simulink model "MotorLink"  (R2020b)
settings: Solver=ode4  StartTime=0.0  StopTime=15  FixedStep=0.001  RelTol=1e-3
values from neighbouring files (symbols this model uses):
  A = [0 1 0; -m*l*g/den -d/den km/den; 0 -ke/L -R/L]    [init_MotorLink.m]
  A_dist = [A_dist; [0 0 0 0]]    [init_MotorLink.m]
  B = [0 0 1/L]'    [init_MotorLink.m]
  B_dist = [B;0]    [init_MotorLink.m]
  C = [1 0 0]    [init_MotorLink.m]
  C_dist = [C,0]    [init_MotorLink.m]
  d = 0.1    [init_MotorLink.m]
  g = 9.81    [init_MotorLink.m]
  h = place(A', C', q)'    [init_MotorLink.m]
  h_dist = place(A_dist', C_dist', q_dist)'    [init_MotorLink.m]
  J = 0.001    [init_MotorLink.m]
  k = kR * inv(T)    [init_MotorLink.m]
  ke = 0.1    [init_MotorLink.m]
  km = 0.1    [init_MotorLink.m]
  L = 0.01    [init_MotorLink.m]
  l = 0.1375    [init_MotorLink.m]
  m = 1    [init_MotorLink.m]
  R = 0.1    [init_MotorLink.m]
settings Model: Creator=baradaran  LastModifiedBy=jsol

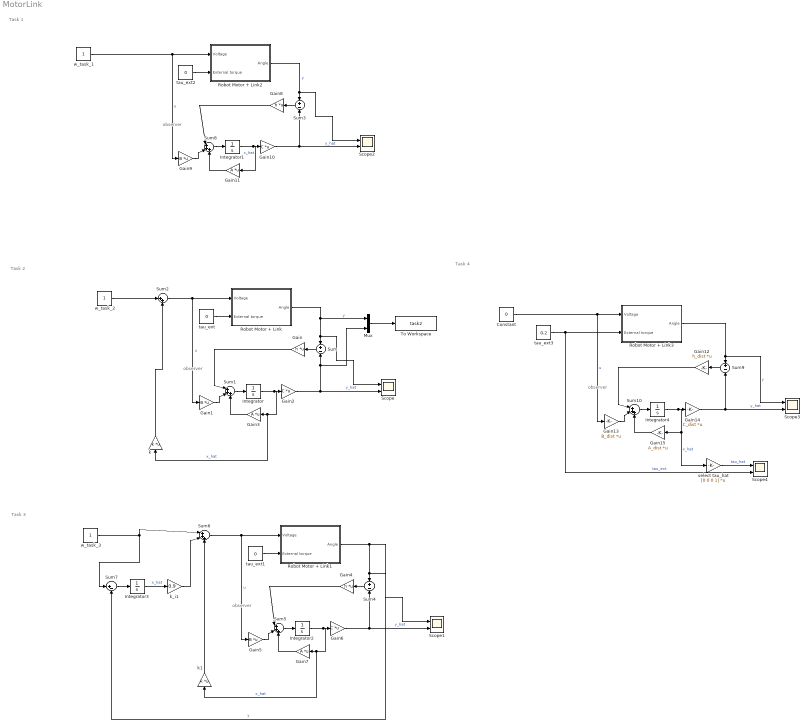
== system MotorLink ==
  note: Task 4
  note: Task 3
  note: Task 2
  note: Task 1
  note: observer
  note: observer
  note: observer
  note: observer
  Constant : Constant  Value=0
  Gain : Gain  Gain=h  Multiplication=Matrix(K*u)
  Gain1 : Gain  Gain=B  Multiplication=Matrix(K*u)
  Gain10 : Gain  Gain=C  Multiplication=Matrix(K*u)
  Gain11 : Gain  Gain=A  Multiplication=Matrix(K*u)
  Gain12 : Gain  Gain=h_dist  Multiplication=Matrix(K*u)
  Gain13 : Gain  Gain=B_dist  Multiplication=Matrix(K*u)
  Gain14 : Gain  Gain=C_dist  Multiplication=Matrix(K*u)
  Gain15 : Gain  Gain=A_dist  Multiplication=Matrix(K*u)
  Gain2 : Gain  Gain=C  Multiplication=Matrix(K*u)
  Gain3 : Gain  Gain=A  Multiplication=Matrix(K*u)
  Gain4 : Gain  Gain=h  Multiplication=Matrix(K*u)
  Gain5 : Gain  Gain=B  Multiplication=Matrix(K*u)
  Gain6 : Gain  Gain=C  Multiplication=Matrix(K*u)
  Gain7 : Gain  Gain=A  Multiplication=Matrix(K*u)
  Gain8 : Gain  Gain=h  Multiplication=Matrix(K*u)
  Gain9 : Gain  Gain=B  Multiplication=Matrix(K*u)
  Integrator{,1..4} (5 alike) : Integrator
  Mux : Mux  Inputs=2
  Robot Motor + Link : Subsystem  mask{J=J, ke=ke, R=R, In=L, km=km, d=d, m=m, l=l, g=g}
      mask prompts: J "Massenträgheitsmoment"; ke "elektrische Motorkonstante"; R "elektrischer Widerstand"; In "Induktivität"; km "mechanische Motorkonstante"; d "mechanische Dämpfung"; m "Gelenkmasse"; l "Massenschwerpunkt des Gelenks"; g "Gravitation"
  Robot Motor + Link1 : Subsystem  mask{J=J, ke=ke, R=R, In=L, km=km, d=d, m=m, l=l, g=g}
      mask prompts: J "Massenträgheitsmoment"; ke "elektrische Motorkonstante"; R "elektrischer Widerstand"; In "Induktivität"; km "mechanische Motorkonstante"; d "mechanische Dämpfung"; m "Gelenkmasse"; l "Massenschwerpunkt des Gelenks"; g "Gravitation"
  Robot Motor + Link2 : Subsystem  mask{J=J, ke=ke, R=R, In=L, km=km, d=d, m=m, l=l, g=g}
      mask prompts: J "Massenträgheitsmoment"; ke "elektrische Motorkonstante"; R "elektrischer Widerstand"; In "Induktivität"; km "mechanische Motorkonstante"; d "mechanische Dämpfung"; m "Gelenkmasse"; l "Massenschwerpunkt des Gelenks"; g "Gravitation"
  Robot Motor + Link3 : Subsystem  mask{J=J, ke=ke, R=R, In=L, km=km, d=d, m=m, l=l, g=g}
      mask prompts: J "Massenträgheitsmoment"; ke "elektrische Motorkonstante"; R "elektrischer Widerstand"; In "Induktivität"; km "mechanische Motorkonstante"; d "mechanische Dämpfung"; m "Gelenkmasse"; l "Massenschwerpunkt des Gelenks"; g "Gravitation"
  Scope{,1..4} (5 alike) : Scope  NumInputPorts=2
  Sum{,3..4,9} (4 alike) : Sum  Inputs=+|-
  Sum{1,5..6,8,10} (5 alike) : Sum  Inputs=|+++
  Sum2 : Sum  Inputs=|++
  Sum7 : Sum  Inputs=|+-
  To Workspace : ToWorkspace  VariableName=task2  SaveFormat=Timeseries  SampleTime=-1
  k : Gain  Gain=k  Multiplication=Matrix(K*u)
  k1 : Gain  Gain=k  Multiplication=Matrix(K*u)
  k_i1 : Gain  Gain=0.9
  select tau_hat : Gain  Gain=[0 0 0 1]  Multiplication=Matrix(K*u)
  tau_ext : Constant  Value=0
  tau_ext1 : Constant  Value=0
  tau_ext2 : Constant  Value=0
  tau_ext3 : Constant  Value=0.2
  w_task_1 : Constant
  w_task_2 : Constant
  w_task_3 : Constant
  wires:
  w_task_2/1 -> Sum2/1
  tau_ext/1 -> Robot Motor + Link/2(External torque)
  Robot Motor + Link/1(Angle) -> Mux/1, Scope/1, Sum/1  "y"
  Gain2/1 -> Scope/2, Mux/2, Sum/2  "y_hat"
  Sum/1 -> Gain/1
  Gain/1 -> Sum1/1
  Gain1/1 -> Sum1/2
  Sum1/1 -> Integrator/1
  Integrator/1 -> k/1, Gain3/1, Gain2/1  "x_hat"
  Gain3/1 -> Sum1/3
  Sum2/1 -> Gain1/1, Robot Motor + Link/1(Voltage)  "u"
  Gain5/1 -> Sum5/2
  Sum4/1 -> Gain4/1
  Gain7/1 -> Sum5/3
  Gain6/1 -> Scope1/2, Sum4/2  "y_hat"
  Sum7/1 -> Integrator3/1
  k1/1 -> Sum6/3
  Integrator2/1 -> k1/1, Gain7/1, Gain6/1  "x_hat"
  Gain4/1 -> Sum5/1
  Robot Motor + Link1/1(Angle) -> Sum7/2, Scope1/1, Sum4/1  "y"
  Sum5/1 -> Integrator2/1
  Integrator3/1 -> k_i1/1  "x_hat"
  w_task_3/1 -> Sum7/1, Sum6/1
  k_i1/1 -> Sum6/2
  tau_ext1/1 -> Robot Motor + Link1/2(External torque)
  Sum6/1 -> Gain5/1, Robot Motor + Link1/1(Voltage)  "u"
  k/1 -> Sum2/2
  Gain9/1 -> Sum8/2
  Sum3/1 -> Gain8/1
  Gain11/1 -> Sum8/3
  Gain10/1 -> Scope2/2, Sum3/2  "y_hat"
  Integrator1/1 -> Gain11/1, Gain10/1  "x_hat"
  Gain8/1 -> Sum8/1
  Sum8/1 -> Integrator1/1
  Robot Motor + Link2/1(Angle) -> Scope2/1, Sum3/1  "y"
  tau_ext2/1 -> Robot Motor + Link2/2(External torque)
  w_task_1/1 -> Gain9/1, Robot Motor + Link2/1(Voltage)  "u"
  tau_ext3/1 -> Robot Motor + Link3/2(External torque), Scope4/2  "tau_ext"
  Gain13/1 -> Sum10/2
  Sum9/1 -> Gain12/1
  Robot Motor + Link3/1(Angle) -> Scope3/1, Sum9/1  "y"
  Constant/1 -> Gain13/1, Robot Motor + Link3/1(Voltage)  "u"
  Gain15/1 -> Sum10/3
  Gain14/1 -> Scope3/2, Sum9/2  "y_hat"
  Integrator4/1 -> select tau_hat/1, Gain15/1, Gain14/1  "x_hat"
  Gain12/1 -> Sum10/1
  Sum10/1 -> Integrator4/1
  select tau_hat/1 -> Scope4/1  "tau_hat"
  Mux/1 -> To Workspace/1

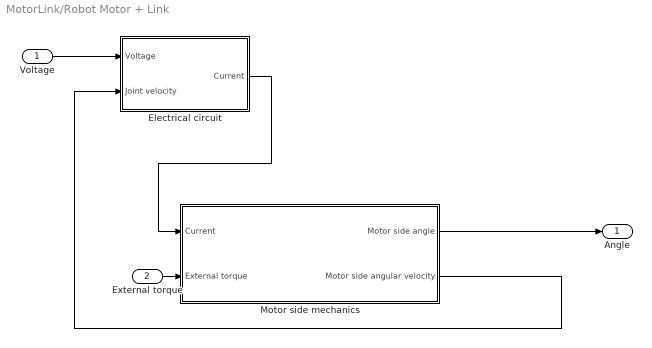
== system MotorLink/Robot Motor + Link ==
  Voltage : Inport
  External torque : Inport  Port=2
  Electrical circuit : Subsystem
  Motor side mechanics : Subsystem
  Angle : Outport  VectorParamsAs1DForOutWhenUnconnected=off
  wires:
  External torque/1 -> Motor side mechanics/2(External torque)
  Motor side mechanics/1(Motor side angle) -> Angle/1
  Motor side mechanics/2(Motor side angular velocity) -> Electrical circuit/2(Joint velocity)
  Electrical circuit/1(Current) -> Motor side mechanics/1(Current)
  Voltage/1 -> Electrical circuit/1(Voltage)

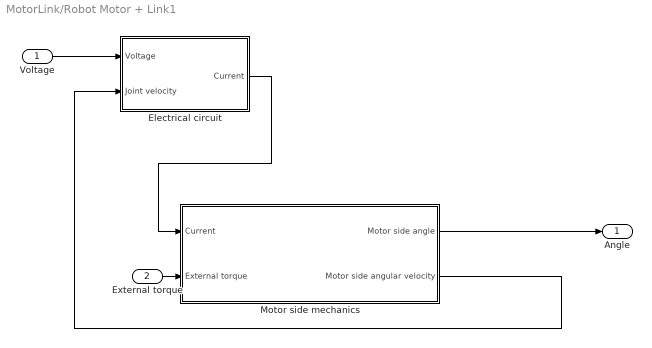
== system MotorLink/Robot Motor + Link1 ==
  Voltage : Inport
  External torque : Inport  Port=2
  Electrical circuit : Subsystem
  Motor side mechanics : Subsystem
  Angle : Outport  VectorParamsAs1DForOutWhenUnconnected=off
  wires:
  External torque/1 -> Motor side mechanics/2(External torque)
  Motor side mechanics/1(Motor side angle) -> Angle/1
  Motor side mechanics/2(Motor side angular velocity) -> Electrical circuit/2(Joint velocity)
  Electrical circuit/1(Current) -> Motor side mechanics/1(Current)
  Voltage/1 -> Electrical circuit/1(Voltage)

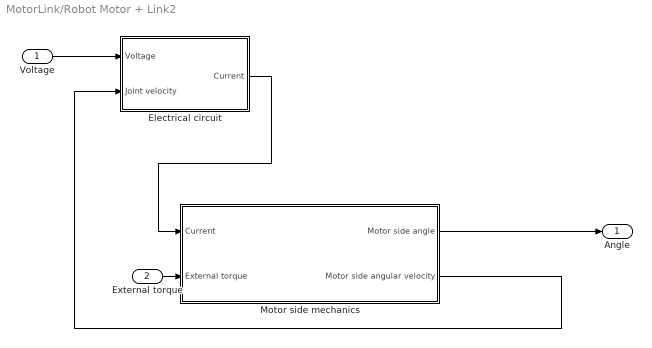
== system MotorLink/Robot Motor + Link2 ==
  Voltage : Inport
  External torque : Inport  Port=2
  Electrical circuit : Subsystem
  Motor side mechanics : Subsystem
  Angle : Outport  VectorParamsAs1DForOutWhenUnconnected=off
  wires:
  External torque/1 -> Motor side mechanics/2(External torque)
  Motor side mechanics/1(Motor side angle) -> Angle/1
  Motor side mechanics/2(Motor side angular velocity) -> Electrical circuit/2(Joint velocity)
  Electrical circuit/1(Current) -> Motor side mechanics/1(Current)
  Voltage/1 -> Electrical circuit/1(Voltage)

== system MotorLink/Robot Motor + Link3 ==
  Voltage : Inport
  External torque : Inport  Port=2
  Electrical circuit : Subsystem
  Motor side mechanics : Subsystem
  Angle : Outport  VectorParamsAs1DForOutWhenUnconnected=off
  wires:
  External torque/1 -> Motor side mechanics/2(External torque)
  Motor side mechanics/1(Motor side angle) -> Angle/1
  Motor side mechanics/2(Motor side angular velocity) -> Electrical circuit/2(Joint velocity)
  Electrical circuit/1(Current) -> Motor side mechanics/1(Current)
  Voltage/1 -> Electrical circuit/1(Voltage)

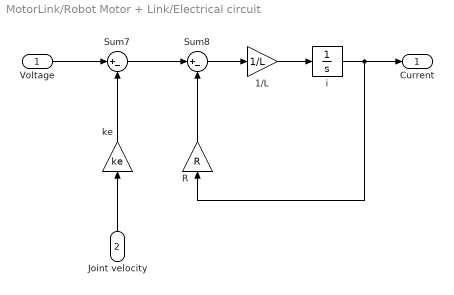
== system MotorLink/Robot Motor + Link/Electrical circuit ==
  Voltage : Inport
  Joint velocity : Inport  Port=2
  1/L : Gain  Gain=1/L
  R : Gain  Gain=R
  Sum7 : Sum  Inputs=|+-
  Sum8 : Sum  Inputs=|+-
  i : Integrator
  ke : Gain  Gain=ke
  Current : Outport  VectorParamsAs1DForOutWhenUnconnected=off
  wires:
  Sum7/1 -> Sum8/1
  i/1 -> R/1, Current/1
  R/1 -> Sum8/2
  Voltage/1 -> Sum7/1
  Joint velocity/1 -> ke/1
  ke/1 -> Sum7/2
  Sum8/1 -> 1/L/1
  1/L/1 -> i/1

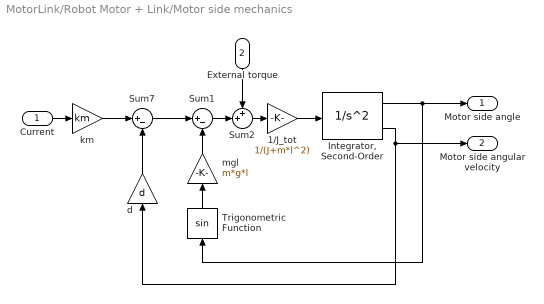
== system MotorLink/Robot Motor + Link/Motor side mechanics ==
  Current : Inport
  External torque : Inport  Port=2
  1/J_tot : Gain  Gain=1/(J+m*l^2)
  "Integrator, Second-Order" : SecondOrderIntegrator
  Sum1 : Sum  Inputs=|+-
  Sum2 : Sum  Inputs=++|
  Sum7 : Sum  Inputs=|+-
  Trigonometric Function : Trigonometry
  d : Gain  Gain=d
  km : Gain  Gain=km
  mgl : Gain  Gain=m*g*l
  Motor side angle : Outport  VectorParamsAs1DForOutWhenUnconnected=off
  Motor side angular velocity : Outport  Port=2  VectorParamsAs1DForOutWhenUnconnected=off
  wires:
  External torque/1 -> Sum2/1
  Sum1/1 -> Sum2/2
  Sum2/1 -> 1/J_tot/1
  Trigonometric Function/1 -> mgl/1
  Current/1 -> km/1
  "Integrator, Second-Order"/2 -> d/1, Motor side angular velocity/1
  1/J_tot/1 -> "Integrator, Second-Order"/1
  "Integrator, Second-Order"/1 -> Motor side angle/1, Trigonometric Function/1
  Sum7/1 -> Sum1/1
  mgl/1 -> Sum1/2
  d/1 -> Sum7/2
  km/1 -> Sum7/1

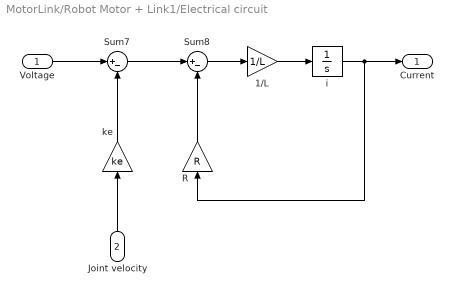
== system MotorLink/Robot Motor + Link1/Electrical circuit ==
  Voltage : Inport
  Joint velocity : Inport  Port=2
  1/L : Gain  Gain=1/L
  R : Gain  Gain=R
  Sum7 : Sum  Inputs=|+-
  Sum8 : Sum  Inputs=|+-
  i : Integrator
  ke : Gain  Gain=ke
  Current : Outport  VectorParamsAs1DForOutWhenUnconnected=off
  wires:
  Sum7/1 -> Sum8/1
  i/1 -> R/1, Current/1
  R/1 -> Sum8/2
  Voltage/1 -> Sum7/1
  Joint velocity/1 -> ke/1
  ke/1 -> Sum7/2
  Sum8/1 -> 1/L/1
  1/L/1 -> i/1

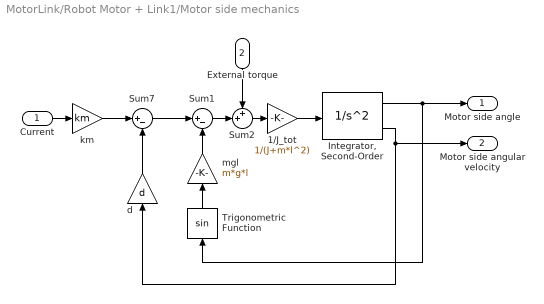
== system MotorLink/Robot Motor + Link1/Motor side mechanics ==
  Current : Inport
  External torque : Inport  Port=2
  1/J_tot : Gain  Gain=1/(J+m*l^2)
  "Integrator, Second-Order" : SecondOrderIntegrator
  Sum1 : Sum  Inputs=|+-
  Sum2 : Sum  Inputs=++|
  Sum7 : Sum  Inputs=|+-
  Trigonometric Function : Trigonometry
  d : Gain  Gain=d
  km : Gain  Gain=km
  mgl : Gain  Gain=m*g*l
  Motor side angle : Outport  VectorParamsAs1DForOutWhenUnconnected=off
  Motor side angular velocity : Outport  Port=2  VectorParamsAs1DForOutWhenUnconnected=off
  wires:
  External torque/1 -> Sum2/1
  Sum1/1 -> Sum2/2
  Sum2/1 -> 1/J_tot/1
  Trigonometric Function/1 -> mgl/1
  Current/1 -> km/1
  "Integrator, Second-Order"/2 -> d/1, Motor side angular velocity/1
  1/J_tot/1 -> "Integrator, Second-Order"/1
  "Integrator, Second-Order"/1 -> Motor side angle/1, Trigonometric Function/1
  Sum7/1 -> Sum1/1
  mgl/1 -> Sum1/2
  d/1 -> Sum7/2
  km/1 -> Sum7/1

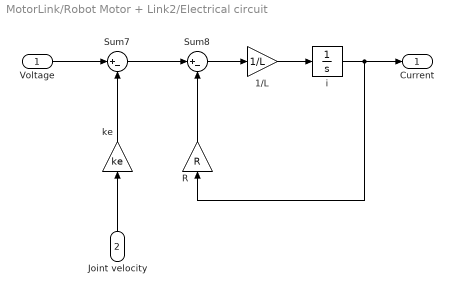
== system MotorLink/Robot Motor + Link2/Electrical circuit ==
  Voltage : Inport
  Joint velocity : Inport  Port=2
  1/L : Gain  Gain=1/L
  R : Gain  Gain=R
  Sum7 : Sum  Inputs=|+-
  Sum8 : Sum  Inputs=|+-
  i : Integrator
  ke : Gain  Gain=ke
  Current : Outport  VectorParamsAs1DForOutWhenUnconnected=off
  wires:
  Sum7/1 -> Sum8/1
  i/1 -> R/1, Current/1
  R/1 -> Sum8/2
  Voltage/1 -> Sum7/1
  Joint velocity/1 -> ke/1
  ke/1 -> Sum7/2
  Sum8/1 -> 1/L/1
  1/L/1 -> i/1

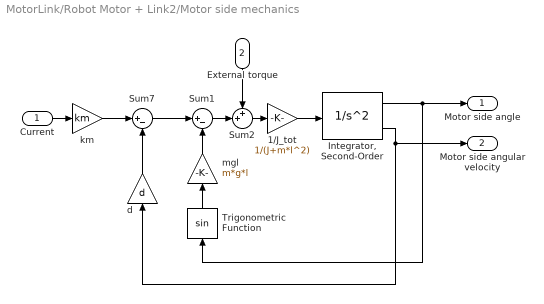
== system MotorLink/Robot Motor + Link2/Motor side mechanics ==
  Current : Inport
  External torque : Inport  Port=2
  1/J_tot : Gain  Gain=1/(J+m*l^2)
  "Integrator, Second-Order" : SecondOrderIntegrator
  Sum1 : Sum  Inputs=|+-
  Sum2 : Sum  Inputs=++|
  Sum7 : Sum  Inputs=|+-
  Trigonometric Function : Trigonometry
  d : Gain  Gain=d
  km : Gain  Gain=km
  mgl : Gain  Gain=m*g*l
  Motor side angle : Outport  VectorParamsAs1DForOutWhenUnconnected=off
  Motor side angular velocity : Outport  Port=2  VectorParamsAs1DForOutWhenUnconnected=off
  wires:
  External torque/1 -> Sum2/1
  Sum1/1 -> Sum2/2
  Sum2/1 -> 1/J_tot/1
  Trigonometric Function/1 -> mgl/1
  Current/1 -> km/1
  "Integrator, Second-Order"/2 -> d/1, Motor side angular velocity/1
  1/J_tot/1 -> "Integrator, Second-Order"/1
  "Integrator, Second-Order"/1 -> Motor side angle/1, Trigonometric Function/1
  Sum7/1 -> Sum1/1
  mgl/1 -> Sum1/2
  d/1 -> Sum7/2
  km/1 -> Sum7/1

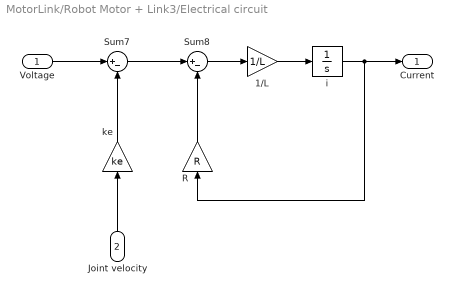
== system MotorLink/Robot Motor + Link3/Electrical circuit ==
  Voltage : Inport
  Joint velocity : Inport  Port=2
  1/L : Gain  Gain=1/L
  R : Gain  Gain=R
  Sum7 : Sum  Inputs=|+-
  Sum8 : Sum  Inputs=|+-
  i : Integrator
  ke : Gain  Gain=ke
  Current : Outport  VectorParamsAs1DForOutWhenUnconnected=off
  wires:
  Sum7/1 -> Sum8/1
  i/1 -> R/1, Current/1
  R/1 -> Sum8/2
  Voltage/1 -> Sum7/1
  Joint velocity/1 -> ke/1
  ke/1 -> Sum7/2
  Sum8/1 -> 1/L/1
  1/L/1 -> i/1

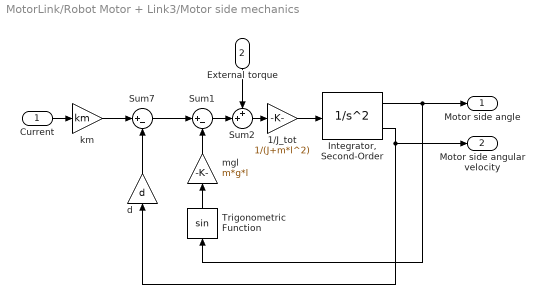
== system MotorLink/Robot Motor + Link3/Motor side mechanics ==
  Current : Inport
  External torque : Inport  Port=2
  1/J_tot : Gain  Gain=1/(J+m*l^2)
  "Integrator, Second-Order" : SecondOrderIntegrator
  Sum1 : Sum  Inputs=|+-
  Sum2 : Sum  Inputs=++|
  Sum7 : Sum  Inputs=|+-
  Trigonometric Function : Trigonometry
  d : Gain  Gain=d
  km : Gain  Gain=km
  mgl : Gain  Gain=m*g*l
  Motor side angle : Outport  VectorParamsAs1DForOutWhenUnconnected=off
  Motor side angular velocity : Outport  Port=2  VectorParamsAs1DForOutWhenUnconnected=off
  wires:
  External torque/1 -> Sum2/1
  Sum1/1 -> Sum2/2
  Sum2/1 -> 1/J_tot/1
  Trigonometric Function/1 -> mgl/1
  Current/1 -> km/1
  "Integrator, Second-Order"/2 -> d/1, Motor side angular velocity/1
  1/J_tot/1 -> "Integrator, Second-Order"/1
  "Integrator, Second-Order"/1 -> Motor side angle/1, Trigonometric Function/1
  Sum7/1 -> Sum1/1
  mgl/1 -> Sum1/2
  d/1 -> Sum7/2
  km/1 -> Sum7/1
